simulink model "MIL4L3_SW6_V1_20220211"  (R2018b)
settings: Solver=FixedStepAuto  StartTime=0.0  StopTime=inf  FixedStep=0.001  RelTol=1e-3
PreLoadFcn:
  | A0_MILtest;
undefined symbols (not defined in the file or in its folder): Clb_ICADirect_LaneDisp_StateFive, Clb_ICADirect_LaneDisp_StateFour, Clb_ICADirect_LaneDisp_StateOne, Clb_ICADirect_LaneDisp_StateThree, Clb_ICADirect_LaneDisp_StateTwo, Clb_ICADirect_LaneDisp_StateZero, Clb_ICADirect_LaneDispSW, Clb_ICADirect_TrnLghtsCom_Switch, Clb_ICADirect_TrnLghtsCom_Value, Clb_ICADirect_TrnLghtsCrtl_Inhb, IMAP_Clb_ACU_Driver_Belt, IMAP_Clb_ACU_Driver_Belt_Over, IMAP_Clb_ACU_Passenger_Belt, IMAP_Clb_ACU_Passenger_Belt_Over, IMAP_Clb_ACU_RearLeft_Belt, IMAP_Clb_ACU_RearLeft_Belt_Over, IMAP_Clb_ACU_RearMiddle_Belt, IMAP_Clb_ACU_RearMiddle_Belt_Over, IMAP_Clb_ACU_RearRight_Belt, IMAP_Clb_ACU_RearRight_Belt_Over, IMAP_Clb_AEB_Switch, IMAP_Clb_AEB_Switch_Over, IMAP_Clb_ALC_TLC_Mode, IMAP_Clb_ALC_TLC_Mode_Over, IMAP_Clb_BCM_Battery_Voltage, IMAP_Clb_BCM_Battery_Voltage_Over, IMAP_Clb_BCM_BrakeLamp_State, IMAP_Clb_BCM_BrakeLamp_State_Over, IMAP_Clb_BCM_CHMSL_Status, IMAP_Clb_BCM_CHMSL_Status_Over, IMAP_Clb_BCM_Door_Lock_State, IMAP_Clb_BCM_Door_Lock_State_Over, IMAP_Clb_BCM_FrontWiper_State, IMAP_Clb_BCM_FrontWiper_State_Over, IMAP_Clb_BCM_FrontWiper_Switch, IMAP_Clb_BCM_FrontWiper_Switch_Over, IMAP_Clb_BCM_HazardLamp, IMAP_Clb_BCM_HazardLamp_Over, IMAP_Clb_BCM_HazardLamp_Switch, IMAP_Clb_BCM_HazardLamp_Switch_Over, IMAP_Clb_BCM_HighBeam_State, IMAP_Clb_BCM_HighBeam_State_Over, IMAP_Clb_BCM_Ignition_State, IMAP_Clb_BCM_Ignition_State_Over, IMAP_Clb_BCM_IHBC_Enabled, IMAP_Clb_BCM_IHBC_Enabled_Over, IMAP_Clb_BCM_Left_Light, IMAP_Clb_BCM_Left_Light_Over, IMAP_Clb_BCM_LeftTurn_Switch, IMAP_Clb_BCM_LeftTurn_Switch_Over, IMAP_Clb_BCM_LF_Door_State, IMAP_Clb_BCM_LF_Door_State_Over, IMAP_Clb_BCM_LowBeam_State, IMAP_Clb_BCM_LowBeam_State_Over, IMAP_Clb_BCM_LR_Door_State, IMAP_Clb_BCM_LR_Door_State_Over, IMAP_Clb_BCM_RF_Door_State, IMAP_Clb_BCM_RF_Door_State_Over, IMAP_Clb_BCM_Right_Light, IMAP_Clb_BCM_Right_Light_Over ... (+547)
libraries: CarMaker4SL x2153, simulink x292, dspstat3 x3, canmsglib x2, simulink_extras x1
(part 33 of 52)

== system MIL4L3_SW6_V1_20220211/CarMaker/VehicleControl/Function/LKA/LKAS1/LL/Fault_Diagnostic ==
  bsInInfo : Inport
  Bus Creator : BusCreator  Inputs=2
  Bus Creator1 : BusCreator  Inputs=10
  Bus Selector3 : BusSelector  OutputSignals=DTC_Indicator.LKAS_BSWDTC_Status
  Bus Selector4 : BusSelector  OutputSignals=bsVehMovInfo.ESC_VehSpd_Valid,bsEPSInfo.EPS_LKA_State,bsEPSInfo.SAS_Clb_State,bsEPSInfo.SAS_Trim_State,bsPTState.TCU_ActualGear,bsEPSInfo.EPS_TrqLim_State,bsEPSInfo.EPS_Trq_State,bsVehMovInfo.ESC_LatAcc_Valid,bsVehMovInfo.ESC_YawRate_Valid,bsVehMovInfo.ESC_LonAcc_Valid
  Compare To Constant26 : simulink/Logic and Bit Operations/Compare To Constant  relop=~=  const=1  OutDataTypeStr=boolean
  Compare To Constant27 : simulink/Logic and Bit Operations/Compare To Constant  relop===  const=4  OutDataTypeStr=boolean
  Compare To Constant29 : simulink/Logic and Bit Operations/Compare To Constant  relop===  const=0  OutDataTypeStr=boolean
  Compare To Constant{30,36..39} (5 alike) : simulink/Logic and Bit Operations/Compare To Constant  relop===  const=1  OutDataTypeStr=boolean
  Compare To Constant34 : simulink/Logic and Bit Operations/Compare To Constant  relop=>  const=3  OutDataTypeStr=boolean
  Compare To Constant35 : simulink/Logic and Bit Operations/Compare To Constant  relop===  const=0  OutDataTypeStr=boolean
  bsSignalFault : Outport
  wires:
  Bus Creator/1 -> bsSignalFault/1
  Bus Selector3/1 -> Bus Creator/1  "<LKAS_BSWDTC_Status>"
  bsInInfo/1 -> Bus Selector4/1, Bus Selector3/1
  Bus Selector4/1 -> Compare To Constant26/1  "<ESC_VehSpd_Valid>"
  Compare To Constant26/1 -> Bus Creator1/1  "Event_FaulVehSpeed"
  Bus Selector4/2 -> Compare To Constant27/1  "<EPS_LKA_State>"
  Bus Selector4/3 -> Compare To Constant29/1  "<SAS_Clb_State>"
  Compare To Constant29/1 -> Bus Creator1/3  "Event_FaulSASClb"
  Bus Selector4/4 -> Compare To Constant30/1  "<SAS_Trim_State>"
  Bus Selector4/5 -> Compare To Constant34/1  "<TCU_ActualGear>"
  Bus Selector4/6 -> Compare To Constant35/1  "<EPS_TrqLim_State>"
  Bus Selector4/7 -> Compare To Constant36/1  "<EPS_Trq_State>"
  Bus Selector4/8 -> Compare To Constant37/1  "<ESC_LatAcc_Valid>"
  Bus Selector4/9 -> Compare To Constant38/1  "<ESC_YawRate_Valid>"
  Bus Selector4/10 -> Compare To Constant39/1  "<ESC_LonAcc_Valid>"
  Compare To Constant30/1 -> Bus Creator1/4  "Event_FaulSASTrim"
  Compare To Constant35/1 -> Bus Creator1/6  "Event_FaulTrqLim"
  Compare To Constant34/1 -> Bus Creator1/5  "Event_FaulTCUGear"
  Compare To Constant36/1 -> Bus Creator1/7  "Event_FaulEPSTrqSt"
  Compare To Constant37/1 -> Bus Creator1/8  "Event_FaulLatAcc"
  Compare To Constant38/1 -> Bus Creator1/9  "Event_FaulYawRate"
  Compare To Constant39/1 -> Bus Creator1/10  "Event_FaulLonAcc"
  Bus Creator1/1 -> Bus Creator/2  "LKAS_ASWDTC_Status"
  Compare To Constant27/1 -> Bus Creator1/2  "Event_FaulEPSLKASt"

== system MIL4L3_SW6_V1_20220211/CarMaker/VehicleControl/Function/LKA/LKAS1/LL/Human Machine Interface (HMI) ==
  HMI_stDACmode : Inport
  HMI_LKA_STATE : Inport  Port=2
  HMI_LDW_STATE : Inport  Port=3
  HMI_LDWWarn : Inport  Port=4
  HMI_R0_Quality : Inport  Port=5
  HMI_L0_Quality : Inport  Port=6
  HMI_EPSInfo : Inport  Port=7
  HMI_camera_common_fault : Inport  Port=8
  HMI_Front_Camera_Blocked : Inport  Port=9
  HMI_bsLLClb : Inport  Port=10
  Bus Creator2 : BusCreator  Inputs=7
  Bus Selector : BusSelector  OutputSignals=bsConstantClb.LKA_SampleTime,bsLLSMConClb.DisblCClb.LL_HandsOff_TextTime,bsLLSMConClb.DisblCClb.LL_HandsOff_WarnTime
  Cast To Single{,1..6} (7 alike) : DataTypeConversion  OutDataTypeStr=uint8
  Ground : Ground
  HMI_Popup_Status : MATLAB Function  TreatAsAtomicUnit=on
  Hands_Off_Warning : MATLAB Function  TreatAsAtomicUnit=on
  LDW_Flag : MATLAB Function  TreatAsAtomicUnit=on
  LDW_Status_Display : MATLAB Function  TreatAsAtomicUnit=on
  LKA_Status_Display : MATLAB Function  TreatAsAtomicUnit=on
  LKA_action_indication : MATLAB Function  TreatAsAtomicUnit=on
  Subsystem : Subsystem
  Vehicle_Lane_Display : MATLAB Function  TreatAsAtomicUnit=on
  HMI_LDWLKA : Outport
  wires:
  Bus Creator2/1 -> HMI_LDWLKA/1
  Hands_Off_Warning/1(Hands_Off_Warning) -> Cast To Single4/1  "Hands_Off_Warning"
  Cast To Single5/1 -> Bus Creator2/6  "LKA_Action_Indication"
  Cast To Single2/1 -> Bus Creator2/3  "LKA_Status_Display"
  LDW_Flag/1(LDW_Flag) -> Cast To Single3/1  "LDW_Flag"
  LDW_Status_Display/1(LDW_Status_Display) -> Cast To Single1/1  "LDW_Status_Display"
  HMI_Popup_Status/1(HMI_Popup_Status) -> Cast To Single6/1  "HMI_Popup_Status"
  Cast To Single1/1 -> Bus Creator2/2  "LDW_Status_Display"
  LKA_Status_Display/1(LKA_Status_Display) -> Cast To Single2/1  "LKA_Status_Display"
  Cast To Single3/1 -> Bus Creator2/4  "LDW_Flag"
  Vehicle_Lane_Display/1(Vehicle_Lane_Display) -> Cast To Single/1  "Vehicle_Lane_Display"
  Cast To Single/1 -> Bus Creator2/1  "Vehicle_Lane_Display"
  Cast To Single6/1 -> Bus Creator2/7  "HMI_Popup_Status"
  LKA_action_indication/1(LKA_Action_Indication) -> Cast To Single5/1  "LKA_Action_Indication"
  Cast To Single4/1 -> Bus Creator2/5  "Hands_Off_Warning"
  HMI_LKA_STATE/1 -> Vehicle_Lane_Display/2(LKA_STATE), LKA_action_indication/2(LKA_STATE), HMI_Popup_Status/2(LKA_STATE), LDW_Flag/2(HMI_LKA_STATE), LKA_Status_Display/2(LKA_STATE), Subsystem/2(LKA_STATE)  "HMI_LKA_STATE"
  HMI_LDW_STATE/1 -> Vehicle_Lane_Display/3(LDW_STATE), LDW_Status_Display/2(LDW_STATE), Subsystem/1(LDW_STATE)  "HMI_LDW_STATE"
  Ground/1 -> HMI_Popup_Status/6(stFaultCSyn)  "HMI_stFaultCSyn"
  HMI_L0_Quality/1 -> Vehicle_Lane_Display/5(L0_Quality)  "HMI_L0_Quality"
  HMI_stDACmode/1 -> Vehicle_Lane_Display/1(stDACmode), LDW_Status_Display/1(stDACmode), LKA_action_indication/1(stDACmode), HMI_Popup_Status/1(stDACmode), LDW_Flag/1(HMI_stDACmode), LKA_Status_Display/1(stDACmode)  "HMI_stDACmode"
  HMI_Front_Camera_Blocked/1 -> HMI_Popup_Status/5(Front_Camera_Blocked)  "HMI_Front_Camera_Blocked"
  HMI_R0_Quality/1 -> Vehicle_Lane_Display/4(R0_Quality)  "HMI_R0_Quality"
  HMI_camera_common_fault/1 -> HMI_Popup_Status/4(camera_common_fault)  "HMI_camera_common_fault"
  HMI_EPSInfo/1 -> Subsystem/3(EPSInfo)  "HMI_EPSInfo"
  Subsystem/2(HandsOff1_Text) -> HMI_Popup_Status/3(HandsOff)
  Subsystem/1(HandsOff2_Warn) -> Hands_Off_Warning/1(HandsOff)
  HMI_LDWWarn/1 -> LDW_Flag/3(HMI_LDWWarnInfo)
  HMI_bsLLClb/1 -> Bus Selector/1  "HMI_bsLLClb"
  Bus Selector/1 -> Subsystem/4(SampleTime)  "<LKA_SampleTime>"
  Bus Selector/2 -> Subsystem/5(HandsOff_Text)  "<LL_HandsOff_TextTime>"
  Bus Selector/3 -> Subsystem/6(HandsOff_Warn)  "<LL_HandsOff_WarnTime>"

== system MIL4L3_SW6_V1_20220211/CarMaker/VehicleControl/Function/LKA/LKAS1/LL/LL Inputs Mapping ==
  bsInInfo : Inport
  bsLLClb : Inport  Port=2
  Bus Creator : BusCreator  Inputs=7
  Bus Selector : BusSelector  OutputSignals=bsMP5Info,bsLaneInfo,bsEPSInfo,bsVehMovInfo,bsSWAInfo,bsBCMInfo,bsPTState
  bsBCMInfo : Subsystem
  bsEPSInfo : Subsystem
  bsLaneInfo : Subsystem
  bsMP5Info : Subsystem
  bsPTState : Subsystem
  bsSWAInfo : Subsystem
  bsVehMovInfo : Subsystem
  bsInfo : Outport
  wires:
  bsSWAInfo/1(bsSWAInfoOut) -> Bus Creator/5  "bsSWAInfo"
  bsLaneInfo/1(bsLaneInfoOut) -> Bus Creator/2  "bsLaneInfo"
  bsPTState/1(bsPTStateOut) -> Bus Creator/7  "bsPTState"
  Bus Selector/7 -> bsPTState/1(bsPTStateIn)  "<bsPTState>"
  bsBCMInfo/1(bsBCMInfoOut) -> Bus Creator/6  "bsBCMInfo"
  bsMP5Info/1(bsMP5InfoOut) -> Bus Creator/1  "bsMP5Info"
  Bus Selector/1 -> bsMP5Info/1(bsMP5InfoIn)  "<bsMP5Info>"
  Bus Selector/6 -> bsBCMInfo/1(bsBCMInfoIn)  "<bsBCMInfo>"
  Bus Selector/5 -> bsSWAInfo/1(bsSWAInfoIn)  "<bsSWAInfo>"
  bsVehMovInfo/1(bsVehMovInfoOut) -> Bus Creator/4  "bsVehMovInfo"
  Bus Selector/4 -> bsVehMovInfo/1(bsVehMovInfoIn)  "<bsVehMovInfo>"
  bsEPSInfo/1(bsEPSInfoOut) -> Bus Creator/3  "bsEPSInfo"
  Bus Selector/3 -> bsEPSInfo/1(bsEPSInfoIn)  "<bsEPSInfo>"
  Bus Selector/2 -> bsLaneInfo/2(bsLaneInfoIn)  "<bsLaneInfo>"
  Bus Creator/1 -> bsInfo/1
  bsInInfo/1 -> Bus Selector/1
  bsLLClb/1 -> bsLaneInfo/1(bsLLClb)

== system MIL4L3_SW6_V1_20220211/CarMaker/VehicleControl/Function/LKA/LKAS1/LL/LLOn ==
  bsInInfo : Inport
  bsLLClb : Inport  Port=2
  bsSignalFault : Inport  Port=3
  Enable : EnablePort  StatesWhenEnabling=reset
      settings: AttributesFormatString=states = %<StatesWhenEnabling>
  LDW : Subsystem  Description=|  TreatAsAtomicUnit=on
      | Block Name: Lane Departure Warning
      | Ab.: LDW
      | No.: 1.3.0.0
      | Rev: 0.0.1
      | Update Date: 19-3-26
  LKA : Subsystem  Description=|  TreatAsAtomicUnit=on
      | Block Name: Lane Keeping Assistance
      | Ab.: LKA
      | No.: 1.2.0.0
      | Rev: 0.0.1
      | Update Date: 19-5-13
  LKA Input Processing (LKAInP) : Subsystem
  LL State Determination (LLStateDet) : Subsystem
  LL_Mon : Subsystem
  bsLLState : Outport  OutputWhenDisabled=reset  InitialOutput=0
      settings: AttributesFormatString=%<OutputWhenDisabled> = %<InitialOutput>
  LDW_Flag : Outport  Port=2  OutputWhenDisabled=reset  InitialOutput=0
      settings: AttributesFormatString=%<OutputWhenDisabled> = %<InitialOutput>
  phiSWACmd : Outport  Port=3  OutputWhenDisabled=reset  InitialOutput=0
      settings: AttributesFormatString=%<OutputWhenDisabled> = %<InitialOutput>
  M : Outport  Port=4  OutputWhenDisabled=reset  InitialOutput=0
      settings: AttributesFormatString=%<OutputWhenDisabled> = %<InitialOutput>
  LLMon : Outport  Port=5
      settings: AttributesFormatString=%<OutputWhenDisabled> = %<InitialOutput>
  wires:
  LL State Determination (LLStateDet)/2(LLStateDet_stLDWActvFlg) -> LDW/Enable
  [bsLLClb] -> LL State Determination (LLStateDet)/3(LLStateDet_bsLLClb)
  [bsLLClb] -> LKA Input Processing (LKAInP)/2(LKAInP_bsLLClb)
  LL State Determination (LLStateDet)/1(LLStateDet_bsLLState) -> bsLLState/1
  [bsLLClb] -> LDW/2(LDW_bsLDWClb)
  LKA Input Processing (LKAInP)/1(LKAInP_bsLKAInPInfo) -> LKA/2(LKA_bsLKAInPInfo), LL State Determination (LLStateDet)/2(LLStateDet_bsLKAInPInfo), LDW/1(LDW_bsLKAInfoSyn)
  bsLLClb/1 -> [bsLLClb]
  LL State Determination (LLStateDet)/3(LLStateDet_stLKAActvFlg) -> LKA/Enable, [ActFlg]
  LDW/1(LDW_Flag) -> LDW_Flag/1  "LDW_Flag"
  bsInInfo/1 -> LKA/1(LKA_bsInInfoSyn), LL State Determination (LLStateDet)/1(LLStateDet_bsInInfoSyn), LKA Input Processing (LKAInP)/1(LKAInP_bsInInfoSyn)
  [ExitFlg] -> LL State Determination (LLStateDet)/4(LLStateDet_stExitFlg)
  LKA/2(LKA_phiSWACmd) -> phiSWACmd/1  "OutputSWACmd"
  LKA/1(LKA_ExitFlg) -> [ExitFlg]
  bsSignalFault/1 -> LL State Determination (LLStateDet)/5(LLStateDet_SignalFault)
  LKA/3(LKA_M) -> M/1  "OutputM"
  LKA/4(LKAMon) -> [LKAMon]
  [LKAMon] -> LL_Mon/2(LKAMon)
  LL_Mon/1(LLMon) -> LLMon/1
  [bsLLClb] -> LKA/3(LKA_bsLKAClb)
  [ActFlg] -> LKA Input Processing (LKAInP)/3(In3)
  LL State Determination (LLStateDet)/4(Disable_Reason) -> LL_Mon/1(Disable_Reason)

== system MIL4L3_SW6_V1_20220211/CarMaker/VehicleControl/Function/LKA/LKAS1/LL/LLOut ==
  LLOut_bsLLState : Inport
  LLOut_phiSWACmd : Inport  Port=2
  LLOut_bsLLHMI : Inport  Port=3
  LLOut_M : Inport  Port=4
  LLOut_bsInfo : Inport  Port=5
  1 : Constant  OutDataTypeStr=uint8
      settings: AttributesFormatString=DT: %<OutDataTypeStr>
  2 : Constant  OutDataTypeStr=uint8
      settings: AttributesFormatString=DT: %<OutDataTypeStr>
  Angle2Trq : Subsystem
  Bus Creator : BusCreator  Inputs=15
  Bus Selector1 : BusSelector  OutputSignals=LKA_State,DACMode
  Bus Selector2 : BusSelector  OutputSignals=Vehicle_Lane_Display,LDW_Status_Display,LKA_Status_Display,LDW_Flag,Hands_Off_Warning,LKA_Action_Indication,HMI_Popup_Status
  Bus Selector3 : BusSelector  OutputSignals=bsSWAInfo.SW_Angle
  Cast To Single : DataTypeConversion  OutDataTypeStr=single
  Cast To Single{1..2,4..12} (11 alike) : DataTypeConversion  OutDataTypeStr=uint8
  Cast To Single13 : DataTypeConversion  OutDataTypeStr=single
  Cast To Single3 : DataTypeConversion  OutDataTypeStr=single
  Compare To Constant : simulink/Logic and Bit Operations/Compare To Constant  relop===  const=4  OutDataTypeStr=boolean
  Compare To Constant1 : simulink/Logic and Bit Operations/Compare To Constant  relop=>  const=0  OutDataTypeStr=boolean
  Compare To Constant2 : simulink/Logic and Bit Operations/Compare To Constant  relop===  const=4  OutDataTypeStr=boolean
  Compare To Constant3 : simulink/Logic and Bit Operations/Compare To Constant  relop===  const=3  OutDataTypeStr=boolean
  Constant1 : Constant  OutDataTypeStr=uint8
  Constant2 : Constant  Value=2  OutDataTypeStr=uint8
  Constant3 : Constant  Value=3  OutDataTypeStr=uint8
  Constant4 : Constant  Value=4  OutDataTypeStr=uint8
  Constant5 : Constant  Value=4  OutDataTypeStr=uint8
  Constant6 : Constant  Value=5  OutDataTypeStr=uint8
  Logical Operator : Logic  Operator=OR  AllPortsSameDT=off  OutDataTypeStr=boolean
  Multiport Switch : MultiPortSwitch  DataPortOrder=Zero-based contiguous  Inputs=7  zeroidx=on
  Switch : Switch  Criteria=u2 ~= 0
      settings: AttributesFormatString=%<Criteria>
  Switch1 : Switch  Criteria=u2 ~= 0
      settings: AttributesFormatString=%<Criteria>
  Switch2 : Switch  Criteria=u2 ~= 0
      settings: AttributesFormatString=%<Criteria>
  x0 : Constant  Value=0  OutDataTypeStr=uint8
      settings: AttributesFormatString=DT: %<OutDataTypeStr>
  x1 : Constant  Value=0  OutDataTypeStr=uint8
      settings: AttributesFormatString=DT: %<OutDataTypeStr>
  x2 : Constant  Value=0  OutDataTypeStr=uint8
      settings: AttributesFormatString=DT: %<OutDataTypeStr>
  LL_bsLLOut : Outport
      settings: AttributesFormatString=Disable Action: %<OutputWhenDisabled>
  wires:
  Cast To Single13/1 -> Bus Creator/15  "LKA_TorqueReq_Value"
  [LKA_TorqueReq_Value] -> Cast To Single13/1  "LKA_TorqueReq_Value"
  Cast To Single1/1 -> Bus Creator/14  "LKA_Torque_Req"
  [LKA_Torque_Req] -> Cast To Single1/1  "LKA_TorqueReq"
  Cast To Single7/1 -> Bus Creator/8  "LKA_Action_Indication"
  Compare To Constant/1 -> Switch/2, Switch1/2
  [Vehicle_Lane_Display] -> Cast To Single12/1  "Vehicle_Lane_Display"
  [EPS_LKA_Control] -> Cast To Single4/1  "EPS_LKA_Control"
  [LDW_Flag] -> Cast To Single5/1  "LDW_Flag"
  [EPS_Factor_Control] -> Cast To Single3/1  "EPS_Factor_Control"
  [LKA_Action_Indication] -> Cast To Single7/1  "LKA_Action_Indication"
  Constant6/1 -> Multiport Switch/8
  Cast To Single5/1 -> Bus Creator/6  "LDW_Flag"
  [HMI_Popup_Status] -> Cast To Single9/1  "HMI_Popup_Status"
  Bus Selector1/1 -> Multiport Switch/1  "<LKA_State>"
  [LKA_Status_Display] -> Cast To Single8/1  "LKA_Status_Display"
  [LKA_SWA_Control] -> Cast To Single/1  "LKA_SWA_Control"
  Cast To Single/1 -> Bus Creator/2  "LKA_SWA_Control"
  [LDW_Status_Display] -> Cast To Single6/1  "LDW_Status_Display"
  [LKA_Switch_State] -> Cast To Single10/1  "LKA_Switch_State"
  [Hands_Off_Warning] -> Cast To Single11/1  "Hands_Off_Warning"
  Cast To Single8/1 -> Bus Creator/9  "LKA_Status_Display"
  Cast To Single4/1 -> Bus Creator/5  "EPS_LKA_Control"
  Cast To Single10/1 -> Bus Creator/11  "LKA_Switch_State"
  Bus Selector1/2 -> Bus Creator/1, Compare To Constant1/1  "<DACMode>"
  Constant2/1 -> Multiport Switch/4
  Cast To Single2/1 -> Bus Creator/3  "EPS_State_Ctl"
  Bus Creator/1 -> LL_bsLLOut/1
  Cast To Single3/1 -> Bus Creator/4  "EPS_Factor_Control"
  Constant3/1 -> Multiport Switch/5
  Multiport Switch/1 -> Compare To Constant2/1, Compare To Constant3/1, [EPS_State_Ctl], Compare To Constant/1  "EPS_State_Ctl"
  Switch/1 -> [EPS_Factor_Control]  "EPS_Factor_Control"
  Cast To Single6/1 -> Bus Creator/7  "LDW_Status_Display"
  Cast To Single12/1 -> Bus Creator/13  "Vehicle_Lane_Display"
  [EPS_State_Ctl] -> Cast To Single2/1  "EPS_State_Ctl"
  LLOut_bsLLState/1 -> Bus Selector1/1
  Compare To Constant1/1 -> [LKA_Switch_State]
  Constant4/1 -> Multiport Switch/6
  Cast To Single9/1 -> Bus Creator/10  "HMI_Popup_Status"
  LLOut_M/1 -> Switch/1
  Cast To Single11/1 -> Bus Creator/12  "Hands_Off_Warning"
  Constant5/1 -> Multiport Switch/7
  Constant1/1 -> Multiport Switch/2, Multiport Switch/3
  Bus Selector2/5 -> [Hands_Off_Warning]  "<Hands_Off_Warning>"
  Bus Selector2/6 -> [LKA_Action_Indication]  "<LKA_Action_Indication>"
  Bus Selector2/2 -> [LDW_Status_Display]  "<LDW_Status_Display>"
  LLOut_bsLLHMI/1 -> Bus Selector2/1
  Bus Selector2/4 -> [LDW_Flag]  "<LDW_Flag>"
  Bus Selector2/3 -> [LKA_Status_Display]  "<LKA_Status_Display>"
  Bus Selector2/7 -> [HMI_Popup_Status]  "<HMI_Popup_Status>"
  Bus Selector2/1 -> [Vehicle_Lane_Display]  "<Vehicle_Lane_Display>"
  Switch1/1 -> [LKA_Torque_Req]  "LKA_Torque_Req"
  1/1 -> Switch1/1
  x0/1 -> Switch1/3
  LLOut_phiSWACmd/1 -> [LKA_SWA_Control]  "LMS_phiSWACmd"
  [LKA_Torque_Req] -> Angle2Trq/1(LKA_Torque_Req)  "LKA_Torque_Req"
  [LKA_SWA_Control] -> Angle2Trq/2(Target_Angle)  "LKA_SWA_Control"
  Angle2Trq/1(torque) -> [LKA_TorqueReq_Value]
  LLOut_bsInfo/1 -> Bus Selector3/1
  Bus Selector3/1 -> Angle2Trq/3(Stearing_Angle)  "<SW_Angle>"
  x1/1 -> Switch/3
  Compare To Constant2/1 -> Logical Operator/1
  Compare To Constant3/1 -> Logical Operator/2
  Logical Operator/1 -> Switch2/2
  Switch2/1 -> [EPS_LKA_Control]  "EPS_LKA_Control"
  2/1 -> Switch2/1
  x2/1 -> Switch2/3

== system MIL4L3_SW6_V1_20220211/CarMaker/VehicleControl/Function/LKA/LKAS1/LLClb/ConstantClb ==
  Bus Creator : BusCreator  Inputs=6
  Data Type Conversion{2..4,6,13,22} (6 alike) : DataTypeConversion  OutDataTypeStr=single
  LKA_CarWidth=1.8 : Constant  Value=LKA_CarWidth
  LKA_SampleTime=0.01 : Constant  Value=LKA_SampleTime  OutDataTypeStr=single
  LKA_StrRatio_C=15.3 : Constant  Value=LKA_StrRatio_C
  LKA_Veh2CamL_C=1.56 : Constant  Value=LKA_Veh2CamL_C
  LKA_Veh2CamW_C=0.9 : Constant  Value=LKA_Veh2CamW_C  OutDataTypeStr=single
  LKA_WhlBaseL_C=2.65 : Constant  Value=LKA_WhlBaseL_C
  Switch{,1..3,11,19} (6 alike) : Switch  Criteria=u2 ~= 0  OutDataTypeStr=single
  ConstantClb : Outport
  wires:
  LKA_SampleTime=0.01/1 -> Switch19/3  "LKA_SampleTime"
  Data Type Conversion3/1 -> Switch19/1, Switch19/2
  Switch19/1 -> Bus Creator/1  "LKA_SampleTime"
  Switch2/1 -> Bus Creator/4  "LKA_WhlBaseL_C"
  Switch/1 -> Bus Creator/2  "LKA_Veh2CamW_C"
  Switch1/1 -> Bus Creator/3  "LKA_Veh2CamL_C"
  Switch11/1 -> Bus Creator/6  "LKA_CarWidth"
  Switch3/1 -> Bus Creator/5  "LKA_StrRatio_C"
  Bus Creator/1 -> ConstantClb/1
  LKA_CarWidth=1.8/1 -> Switch11/3  "LKA_CarWidth"
  Data Type Conversion22/1 -> Switch11/2, Switch11/1
  LKA_StrRatio_C=15.3/1 -> Switch3/3  "LKA_StrRatio_C"
  Data Type Conversion6/1 -> Switch3/2, Switch3/1
  Data Type Conversion4/1 -> Switch2/2, Switch2/1
  LKA_WhlBaseL_C=2.65/1 -> Switch2/3  "LKA_WhlBaseL_C"
  LKA_Veh2CamL_C=1.56/1 -> Switch1/3  "LKA_Veh2CamL_C"
  Data Type Conversion2/1 -> Switch1/2, Switch1/1
  Data Type Conversion13/1 -> Switch/2, Switch/1
  LKA_Veh2CamW_C=0.9/1 -> Switch/3  "LKA_Veh2CamW_C"

== system MIL4L3_SW6_V1_20220211/CarMaker/VehicleControl/Function/LKA/LKAS1/LLClb/LDWClb ==
  Bus Creator : BusCreator  Inputs=1
  Data Type Conversion6 : DataTypeConversion  OutDataTypeStr=single
  LL_LDWS_SUPPRESS_HEADING=2 : Constant  Value=LL_LDWS_SUPPRESS_HEADING  OutDataTypeStr=single
  Switch2 : Switch  Criteria=u2 ~= 0  OutDataTypeStr=single
  LDWClb : Outport
  wires:
  Data Type Conversion6/1 -> Switch2/2, Switch2/1
  LL_LDWS_SUPPRESS_HEADING=2/1 -> Switch2/3
  Switch2/1 -> Bus Creator/1  "LL_LDWS_SUPPRESS_HEADING"
  Bus Creator/1 -> LDWClb/1

== system MIL4L3_SW6_V1_20220211/CarMaker/VehicleControl/Function/LKA/LKAS1/LLClb/LKAClb ==
  Bus Creator : BusCreator  Inputs=16
  Bus Creator2 : BusCreator  Inputs=16
  Bus Creator3 : BusCreator  Inputs=11
  Bus Creator4 : BusCreator  Inputs=5
  Data Type Conversion{1..34,36..38,49..50,52..55} (43 alike) : DataTypeConversion  OutDataTypeStr=single
  Data Type Conversion35 : DataTypeConversion  OutDataTypeStr=boolean
  Data Type Conversion47 : DataTypeConversion  OutDataTypeStr=boolean
  LL_CompHdAg_C=0.005 : Constant  Value=LL_CompHdAg_C  OutDataTypeStr=single
  LL_CompSWA_C=0 : Constant  Value=LL_CompSWA_C  OutDataTypeStr=single
  LL_CrvtPrvwT_C=0.45 : Constant  Value=LL_CrvtPrvwT_C  OutDataTypeStr=single
  LL_DesDvt_C=0.2 : Constant  Value=LL_DesDvt_C  OutDataTypeStr=single
  LL_DvtComp_C=0 : Constant  Value=LL_DvtComp_C  OutDataTypeStr=single
  LL_DvtPrvwT_C=0.45 : Constant  Value=LL_DvtPrvwT_C  OutDataTypeStr=single
  LL_HdAgExT_C=15 : Constant  Value=LL_HdAgExT_C  OutDataTypeStr=single
  LL_HdAgPrvwT_C=0.45 : Constant  Value=LL_HdAgPrvwT_C  OutDataTypeStr=single
  LL_LAccMax_C=3 : Constant  Value=LL_LAccMax_C  OutDataTypeStr=single
  LL_LAccRMax_C=5 : Constant  Value=LL_LAccRMax_C  OutDataTypeStr=single
  LL_LFClb_TFC_FfCtlRatio_C=1 : Constant  Value=LL_LFClb_TFC_FfCtlRatio_C  OutDataTypeStr=single
  LL_LFClb_TFC_KdBalance_C=1.2 : Constant  Value=LL_LFClb_TFC_KdBalance_C  OutDataTypeStr=single
  LL_LFClb_TFC_KdMaxSWA_C=20 : Constant  Value=LL_LFClb_TFC_KdMaxSWA_C  OutDataTypeStr=single
  LL_LFClb_TFC_KdV1_C=250 : Constant  Value=LL_LFClb_TFC_KdV1_C  OutDataTypeStr=single
  LL_LFClb_TFC_KdV2_C=250 : Constant  Value=LL_LFClb_TFC_KdV2_C  OutDataTypeStr=single
  LL_LFClb_TFC_KdVehSpdLwr_C=60 : Constant  Value=LL_LFClb_TFC_KdVehSpdLwr_C  OutDataTypeStr=single
  LL_LFClb_TFC_KdVehSpdUpr_C=120 : Constant  Value=LL_LFClb_TFC_KdVehSpdUpr_C  OutDataTypeStr=single
  LL_LFClb_TFC_KiMaxSWA_C=5 : Constant  Value=LL_LFClb_TFC_KiMaxSWA_C  OutDataTypeStr=single
  LL_LFClb_TFC_Ki_C=0.01 : Constant  Value=LL_LFClb_TFC_Ki_C  OutDataTypeStr=single
  LL_LFClb_TFC_KpKlat_C=-4.5 : Constant  Value=LL_LFClb_TFC_KpKlat_C  OutDataTypeStr=single
  LL_LFClb_TFC_KpV1_C=40 : Constant  Value=LL_LFClb_TFC_KpV1_C  OutDataTypeStr=single
  LL_LFClb_TFC_KpV2_C=40 : Constant  Value=LL_LFClb_TFC_KpV2_C  OutDataTypeStr=single
  LL_LFClb_TFC_KpVehSpdLwr_C=60 : Constant  Value=LL_LFClb_TFC_KpVehSpdLwr_C  OutDataTypeStr=single
  LL_LFClb_TFC_KpVehSpdUpr_C=120 : Constant  Value=LL_LFClb_TFC_KpVehSpdUpr_C  OutDataTypeStr=single
  LL_LFClb_TFC_Kp_C=1 : Constant  Value=LL_LFClb_TFC_Kp_C  OutDataTypeStr=single
  LL_LFClb_TFC_PrvwT_C=2 : Constant  Value=LL_LFClb_TFC_PrvwT_C  OutDataTypeStr=single
  LL_LKAExPrcs_ExitC0Dvt=0.01 : Constant  Value=LL_LKAExPrcs_ExitC0Dvt  OutDataTypeStr=single
  LL_LKAExPrcs_ExitC0Swt=1 : Constant  Value=LL_LKAExPrcs_ExitC0Swt  OutDataTypeStr=boolean
  LL_LKAExPrcs_tiExitTime3=0.2 : Constant  Value=LL_LKAExPrcs_tiExitTime3  OutDataTypeStr=single
  LL_LKAExPrcs_tiExitTime3=4 : Constant  Value=LL_LKAExPrcs_tiExitTime2  OutDataTypeStr=single
  LL_LKAExPrcs_tiExitTime3=8 : Constant  Value=LL_LKAExPrcs_tiExitTime1  OutDataTypeStr=single
  LL_LKASWASyn_M0=0.4 : Constant  Value=LL_LKASWASyn_M0  OutDataTypeStr=single
  LL_LKASWASyn_M1=0.8 : Constant  Value=LL_LKASWASyn_M1  OutDataTypeStr=single
  LL_LKASWASyn_M2=0.3 : Constant  Value=LL_LKASWASyn_M2  OutDataTypeStr=single
  LL_LKASWASyn_M3K=0.2 : Constant  Value=LL_LKASWASyn_M3K  OutDataTypeStr=single
  LL_LKASWASyn_SWAaddMax=8 : Constant  Value=LL_LKASWASyn_SWAaddMax  OutDataTypeStr=single
  LL_LKASWASyn_T2=4 : Constant  Value=LL_LKASWASyn_T2  OutDataTypeStr=single
  LL_LKASWASyn_TrqMax=1.5 : Constant  Value=LL_LKASWASyn_TrqMax  OutDataTypeStr=single
  LL_LKASWASyn_TrqSwaAddSwt=1 : Constant  Value=LL_LKASWASyn_TrqSwaAddSwt  OutDataTypeStr=boolean
  LL_LKASWASyn_TrqSwaRateDiff=-0.2 : Constant  Value=LL_LKASWASyn_TrqSwaRateDiff  OutDataTypeStr=single
  LL_LKASWASyn_tiTrqSwaRtTime=0.2 : Constant  Value=LL_LKASWASyn_tiTrqSwaRtTime  OutDataTypeStr=single
  LL_LKASWASyn_tiTrqSwaTime=0.3 : Constant  Value=LL_LKASWASyn_tiTrqSwaTime  OutDataTypeStr=single
  LL_LSpdCompT_C=0.4 : Constant  Value=LL_LSpdCompT_C  OutDataTypeStr=single
  LL_NomTAhd_C=0.2 : Constant  Value=LL_NomTAhd_C  OutDataTypeStr=single
  LL_lStpLngth_C=5 : Constant  Value=LL_lStpLngth_C  OutDataTypeStr=single
  Switch{1..24,30..36,39..40,42..45,49..50,52..55} (43 alike) : Switch  Criteria=u2 ~= 0  OutDataTypeStr=single
  Switch46 : Switch  Criteria=u2 ~= 0  OutDataTypeStr=boolean
  Switch47 : Switch  Criteria=u2 ~= 0  OutDataTypeStr=boolean
  LKAClb : Outport
  wires:
  [LLL_LKASWASyn_M3K] -> Data Type Conversion25/1
  Switch18/1 -> Bus Creator3/11  "LL_LKASWASyn_M3K"
  LL_LKASWASyn_M3K=0.2/1 -> Switch18/3
  Data Type Conversion25/1 -> Switch18/1, Switch18/2
  [LLL_LKASWASyn_M0] -> Data Type Conversion12/1
  Switch11/1 -> Bus Creator3/7  "LL_LKASWASyn_M0"
  LL_LKASWASyn_M0=0.4/1 -> Switch11/3
  Data Type Conversion12/1 -> Switch11/1, Switch11/2
  Data Type Conversion19/1 -> Switch13/2, Switch13/1
  LL_LKASWASyn_M1=0.8/1 -> Switch13/3
  Switch13/1 -> Bus Creator3/8  "LL_LKASWASyn_M1"
  [LLL_LKASWASyn_M1] -> Data Type Conversion19/1
  [LLL_LKASWASyn_M2] -> Data Type Conversion20/1
  Switch14/1 -> Bus Creator3/9  "LL_LKASWASyn_M2"
  LL_LKASWASyn_M2=0.3/1 -> Switch14/3
  Data Type Conversion20/1 -> Switch14/1, Switch14/2
  Data Type Conversion24/1 -> Switch16/2, Switch16/1
  LL_LKASWASyn_T2=4/1 -> Switch16/3
  Switch16/1 -> Bus Creator3/10  "LL_LKASWASyn_T2"
  [LLL_LKASWASyn_T2] -> Data Type Conversion24/1
  Data Type Conversion9/1 -> Switch9/2, Switch9/1
  LL_LFClb_TFC_KdBalance_C=1.2/1 -> Switch9/3
  Switch9/1 -> Bus Creator2/16  "LL_LFClb_TFC_KdBalance_C"
  LL_LKAExPrcs_tiExitTime3=8/1 -> Switch55/3
  Data Type Conversion55/1 -> Switch55/1, Switch55/2
  Switch55/1 -> Bus Creator4/1  "LL_LKAExPrcs_tiExitTime1"
  Switch54/1 -> Bus Creator4/2  "LL_LKAExPrcs_tiExitTime2"
  Data Type Conversion54/1 -> Switch54/2, Switch54/1
  LL_LKAExPrcs_tiExitTime3=4/1 -> Switch54/3
  Switch53/1 -> Bus Creator3/6  "LL_LKASWASyn_TrqSwaRateDiff"
  LL_LKASWASyn_TrqSwaRateDiff=-0.2/1 -> Switch53/3
  Data Type Conversion53/1 -> Switch53/1, Switch53/2
  Data Type Conversion52/1 -> Switch52/2, Switch52/1
  LL_LKASWASyn_tiTrqSwaRtTime=0.2/1 -> Switch52/3
  Switch52/1 -> Bus Creator3/5  "LL_LKASWASyn_tiTrqSwaRtTime"
  Switch50/1 -> Bus Creator3/4  "LL_LKASWASyn_tiTrqSwaTime"
  LL_LKASWASyn_tiTrqSwaTime=0.3/1 -> Switch50/3
  Data Type Conversion50/1 -> Switch50/1, Switch50/2
  Data Type Conversion49/1 -> Switch49/2, Switch49/1
  LL_LFClb_TFC_KdMaxSWA_C=20/1 -> Switch49/3
  Switch49/1 -> Bus Creator2/11  "LL_LFClb_TFC_KdMaxSWA_C"
  Data Type Conversion47/1 -> Switch47/2, Switch47/1
  LL_LKASWASyn_TrqSwaAddSwt=1/1 -> Switch47/3
  Switch47/1 -> Bus Creator3/3  "LL_LKASWASyn_TrqSwaAddSwt"
  Switch46/1 -> Bus Creator4/5  "LL_LKAExPrcs_ExitC0Swt"
  LL_LKAExPrcs_ExitC0Swt=1/1 -> Switch46/3
  Data Type Conversion35/1 -> Switch46/1, Switch46/2
  Bus Creator4/1 -> Bus Creator/16  "LL_LKAExPrcs"
  Data Type Conversion33/1 -> Switch44/2, Switch44/1
  LL_LKAExPrcs_ExitC0Dvt=0.01/1 -> Switch44/3
  LL_LKAExPrcs_tiExitTime3=0.2/1 -> Switch45/3
  Data Type Conversion34/1 -> Switch45/1, Switch45/2
  Switch45/1 -> Bus Creator4/3  "LL_LKAExPrcs_tiExitTime3"
  Switch44/1 -> Bus Creator4/4  "LL_LKAExPrcs_ExitC0Dvt"
  Bus Creator3/1 -> Bus Creator/15  "LL_LKASWAClb"
  Switch42/1 -> Bus Creator3/2  "LL_LKASWASyn_TrqMax"
  Switch43/1 -> Bus Creator3/1  "LL_LKASWASyn_SWAaddMax"
  Data Type Conversion32/1 -> Switch43/2, Switch43/1
  LL_LKASWASyn_SWAaddMax=8/1 -> Switch43/3
  LL_LKASWASyn_TrqMax=1.5/1 -> Switch42/3
  Data Type Conversion31/1 -> Switch42/1, Switch42/2
  Data Type Conversion29/1 -> Switch40/2, Switch40/1
  LL_LFClb_TFC_Ki_C=0.01/1 -> Switch40/3
  Data Type Conversion28/1 -> Switch39/2, Switch39/1
  LL_LFClb_TFC_KiMaxSWA_C=5/1 -> Switch39/3
  Switch39/1 -> Bus Creator2/9  "LL_LFClb_TFC_KiMaxSWA_C"
  Switch40/1 -> Bus Creator2/10  "LL_LFClb_TFC_Ki_C"
  Switch36/1 -> Bus Creator2/8  "LL_LFClb_TFC_FfCtlRatio_C"
  Data Type Conversion18/1 -> Switch36/2, Switch36/1
  LL_LFClb_TFC_FfCtlRatio_C=1/1 -> Switch36/3
  LL_LFClb_TFC_KpKlat_C=-4.5/1 -> Switch30/3
  LL_LFClb_TFC_KpVehSpdUpr_C=120/1 -> Switch34/3
  Data Type Conversion14/1 -> Switch31/1, Switch31/2
  LL_LFClb_TFC_KpV2_C=40/1 -> Switch35/3
  Data Type Conversion17/1 -> Switch35/1, Switch35/2
  Data Type Conversion15/1 -> Switch32/1, Switch32/2
  Data Type Conversion4/1 -> Switch34/1, Switch34/2
  Data Type Conversion7/1 -> Switch33/1, Switch33/2
  Data Type Conversion11/1 -> Switch30/1, Switch30/2
  LL_LFClb_TFC_PrvwT_C=2/1 -> Switch32/3
  LL_LFClb_TFC_KpVehSpdLwr_C=60/1 -> Switch31/3
  LL_LFClb_TFC_KpV1_C=40/1 -> Switch33/3
  Switch32/1 -> Bus Creator2/2  "LL_LFClb_TFC_PrvwT_C"
  Switch33/1 -> Bus Creator2/5  "LL_LFClb_TFC_KpV1_C"
  Switch34/1 -> Bus Creator2/4  "LL_LFClb_TFC_KpVehSpdUpr_C"
  Switch31/1 -> Bus Creator2/3  "LL_LFClb_TFC_KpVehSpdLwr_C"
  Switch30/1 -> Bus Creator2/1  "LL_LFClb_TFC_KpKlat_C"
  Switch35/1 -> Bus Creator2/6  "LL_LFClb_TFC_KpV2_C"
  Bus Creator2/1 -> Bus Creator/14  "LL_TFCClb"
  LL_CompSWA_C=0/1 -> Switch17/3
  LL_NomTAhd_C=0.2/1 -> Switch12/3
  LL_lStpLngth_C=5/1 -> Switch15/3
  LL_DesDvt_C=0.2/1 -> Switch10/3
  Data Type Conversion2/1 -> Switch17/1, Switch17/2
  Data Type Conversion22/1 -> Switch10/1, Switch10/2
  Data Type Conversion23/1 -> Switch12/1, Switch12/2
  Data Type Conversion21/1 -> Switch15/1, Switch15/2
  LL_LAccMax_C=3/1 -> Switch7/3
  Data Type Conversion5/1 -> Switch7/1, Switch7/2
  Data Type Conversion10/1 -> Switch4/2, Switch4/1
  LL_LAccRMax_C=5/1 -> Switch4/3
  LL_LSpdCompT_C=0.4/1 -> Switch5/3
  Data Type Conversion13/1 -> Switch5/1, Switch5/2
  Data Type Conversion6/1 -> Switch6/1, Switch6/2
  LL_HdAgExT_C=15/1 -> Switch6/3
  LL_HdAgPrvwT_C=0.45/1 -> Switch3/3
  Data Type Conversion3/1 -> Switch3/1, Switch3/2
  Data Type Conversion16/1 -> Switch2/1, Switch2/2
  LL_CrvtPrvwT_C=0.45/1 -> Switch2/3
  LL_DvtComp_C=0/1 -> Switch1/3
  Data Type Conversion1/1 -> Switch1/1, Switch1/2
  Data Type Conversion8/1 -> Switch8/2, Switch8/1
  LL_DvtPrvwT_C=0.45/1 -> Switch8/3
  Switch12/1 -> Bus Creator/12  "LL_NomTAhd_C"
  Switch10/1 -> Bus Creator/10  "LL_DesDvt_C"
  Switch15/1 -> Bus Creator/11  "LL_lStpLngth_C"
  Switch2/1 -> Bus Creator/5  "LL_CrvtPrvwT_C"
  Switch5/1 -> Bus Creator/9  "LL_LSpdCompT_C"
  Switch4/1 -> Bus Creator/7  "LL_LAccRMax_C"
  Switch7/1 -> Bus Creator/6  "LL_LAccMax_C"
  Switch6/1 -> Bus Creator/8  "LL_HdAgExT_C"
  Switch17/1 -> Bus Creator/13  "LL_CompSWA_C"
  Switch3/1 -> Bus Creator/4  "LL_HdAgPrvwT_C"
  Switch1/1 -> Bus Creator/3  "LL_DvtComp_C"
  Switch8/1 -> Bus Creator/2  "LL_DvtPrvwT_C"
  Bus Creator/1 -> LKAClb/1
  Data Type Conversion26/1 -> Switch19/1, Switch19/2
  Switch19/1 -> Bus Creator2/7  "LL_LFClb_TFC_Kp_C"
  LL_LFClb_TFC_Kp_C=1/1 -> Switch19/3
  Data Type Conversion30/1 -> Switch23/1, Switch23/2
  Switch21/1 -> Bus Creator2/14  "LL_LFClb_TFC_KdV1_C"
  LL_LFClb_TFC_KdVehSpdLwr_C=60/1 -> Switch20/3
  LL_LFClb_TFC_KdV1_C=250/1 -> Switch21/3
  Data Type Conversion36/1 -> Switch22/1, Switch22/2
  Data Type Conversion27/1 -> Switch20/1, Switch20/2
  Switch22/1 -> Bus Creator2/13  "LL_LFClb_TFC_KdVehSpdUpr_C"
  Switch20/1 -> Bus Creator2/12  "LL_LFClb_TFC_KdVehSpdLwr_C"
  LL_LFClb_TFC_KdVehSpdUpr_C=120/1 -> Switch22/3
  Switch23/1 -> Bus Creator2/15  "LL_LFClb_TFC_KdV2_C"
  LL_LFClb_TFC_KdV2_C=250/1 -> Switch23/3
  Data Type Conversion37/1 -> Switch21/1, Switch21/2
  Switch24/1 -> Bus Creator/1  "LL_CompHdAg_C"
  Data Type Conversion38/1 -> Switch24/2, Switch24/1
  LL_CompHdAg_C=0.005/1 -> Switch24/3
